simulink model "IntelligentFan_ClosedLoop"  (R2024b)
settings: Solver=ode15s  StartTime=0.0  StopTime=48  MaxStep=0.05  RelTol=1e-3
values from neighbouring files (symbols this model uses):
  tau_motor_hr = tau_motor/3600    (= 4.33333333333e-05)    [build_closed_loop_model.m]
libraries: fuzblock x1
settings Model: Creator=hasan  LastModifiedBy=hasan

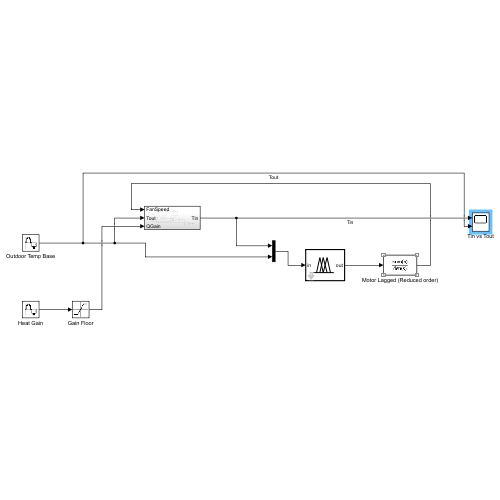
[thumbnail: Simulink's stored preview of the top-level diagram]
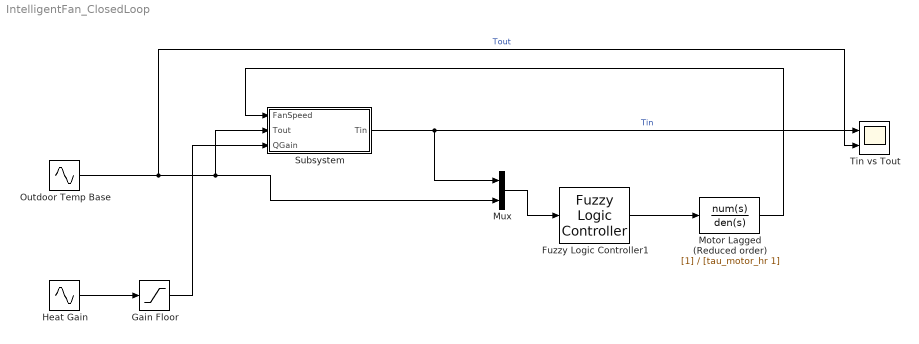
== system IntelligentFan_ClosedLoop ==
  Fuzzy Logic Controller1 : fuzblock/Fuzzy Logic  Controller  FIS='myflcc.fis'  OutputSampleNumber=101  DataType=double  FuzzifiedInputs=off  RuleFiringStrengths=off  RuleOutputs=off  AggregatedOutputs=off  SimulateUsing=Interpreted execution  OutOfRangeInputValueMessage=warning  NoRuleFiredMessage=warning  EmptyOutputFuzzySetMessage=warning
  Gain Floor : Saturate  UpperLimit=700  LowerLimit=300
  Heat Gain : Sin  Amplitude=250  Bias=300  Frequency=2*pi/24  Phase=- 2*pi*8/24  SampleTime=1
  Motor Lagged (Reduced order) : TransferFcn  Denominator=[tau_motor_hr 1]
  Mux : Mux  Inputs=2
  Outdoor Temp Base : Sin  Amplitude=8  Bias=22  Frequency=2*pi/24  Phase=-pi/2 - 2*pi*9/24  SampleTime=1
  Subsystem : Subsystem
  Tin vs Tout : Scope  NumInputPorts=2
  wires:
  Subsystem/1(Tin) -> Tin vs Tout/1, Mux/1  "Tin"
  Mux/1 -> Fuzzy Logic Controller1/1
  Outdoor Temp Base/1 -> Tin vs Tout/2, Subsystem/2(Tout), Mux/2  "Tout"
  Heat Gain/1 -> Gain Floor/1
  Fuzzy Logic Controller1/1 -> Motor Lagged (Reduced order)/1
  Motor Lagged (Reduced order)/1 -> Subsystem/1(FanSpeed)
  Gain Floor/1 -> Subsystem/3(QGain)

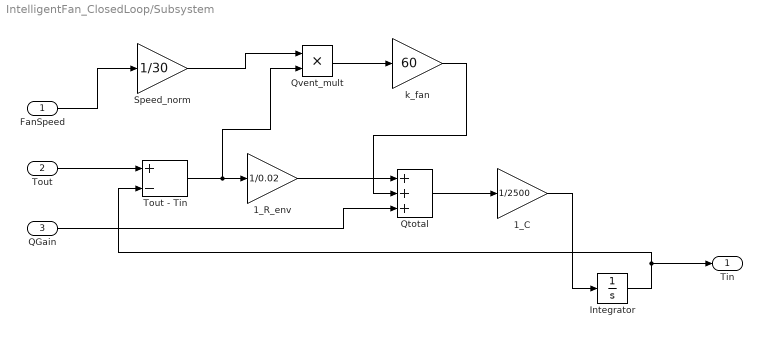
== system IntelligentFan_ClosedLoop/Subsystem ==
  FanSpeed : Inport
  Tout : Inport  Port=2
  QGain : Inport  Port=3
  1_C : Gain  Gain=1/2500
  1_R_env : Gain  Gain=1/0.02
  Integrator : Integrator  InitialCondition=24
  Qtotal : Sum  Inputs=+++
  Qvent_mult : Product
  Speed_norm : Gain  Gain=1/30
  Tout - Tin : Sum  Inputs=+-
  k_fan : Gain  Gain=60
  Tin : Outport
  wires:
  Tout/1 -> Tout - Tin/1
  1_C/1 -> Integrator/1
  Integrator/1 -> Tin/1, Tout - Tin/2
  FanSpeed/1 -> Speed_norm/1
  Speed_norm/1 -> Qvent_mult/1
  Tout - Tin/1 -> Qvent_mult/2, 1_R_env/1
  Qvent_mult/1 -> k_fan/1
  1_R_env/1 -> Qtotal/1
  k_fan/1 -> Qtotal/2
  QGain/1 -> Qtotal/3
  Qtotal/1 -> 1_C/1
